simulink model "Compensator"  (R2013a)
settings: Solver=ode4  StartTime=0.0  StopTime=20.0  FixedStep=0.01  RelTol=1e-3
undefined symbols (not defined in the file): A, Ac, B, Bc, C, Fc, Gc
settings Model: Creator=catalin  LastModifiedBy=catalin

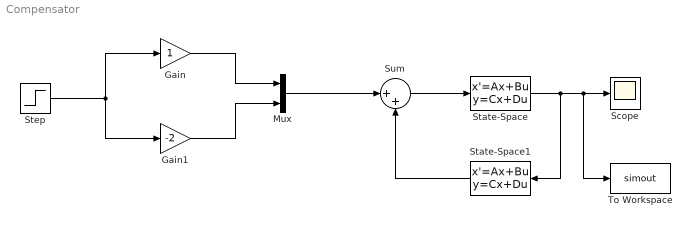
== system Compensator ==
  Gain : Gain
  Gain1 : Gain  Gain=-2
  Mux : Mux  Inputs=2
  Scope : Scope
  State-Space : StateSpace  A=A  B=B  C=C  D=[0,0]
  State-Space1 : StateSpace  A=Ac  B=Bc  C=Fc  D=Gc
  Step : Step  SampleTime=0
  Sum : Sum  Inputs=|++
  To Workspace : ToWorkspace  VariableName=simout  SampleTime=-1  SaveFormat=Timeseries
  wires:
  Step/1 -> Gain/1, Gain1/1
  Gain/1 -> Mux/1
  Gain1/1 -> Mux/2
  Mux/1 -> Sum/1
  Sum/1 -> State-Space/1
  State-Space/1 -> State-Space1/1, To Workspace/1, Scope/1
  State-Space1/1 -> Sum/2
